simulink model "lecture8_simple"  (Simulink 7.1)
settings: Solver=FixedStepDiscrete  StartTime=0.0  StopTime=10.0  RelTol=1e-3
settings Model: Creator=pit  LastModifiedBy=pit

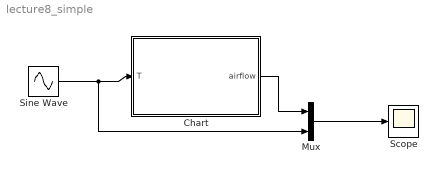
== system lecture8_simple ==
  Chart : Stateflow chart
  Mux : Mux  Inputs=2
  Scope : Scope
  Sine Wave : Sin  Amplitude=50  SampleTime=0
  wires:
  Sine Wave/1 -> Chart/1(T), Mux/2
  Chart/1(airflow) -> Mux/1
  Mux/1 -> Scope/1

== stateflow chart Chart ==
  state Off
    during: airflow=0
  state On
    during:airflow=1
  Off -> On : [T < 10]
  On -> Off : [T > 20]
  (default) -> Off
  data: airflow output double; T input double
